simulink model "TwoDofPassengerCarModel"  (R2021b)
settings: Solver=VariableStepAuto  StartTime=0.0  StopTime=30  RelTol=1e-3
PreLoadFcn:
  | clearvars;
  | M1=300;
  | M2=30;
  | K1=10000;
  | K2=50000;
  | b1=100;
  | b2=30000;
settings Model: Creator=adish  LastModifiedBy=adish

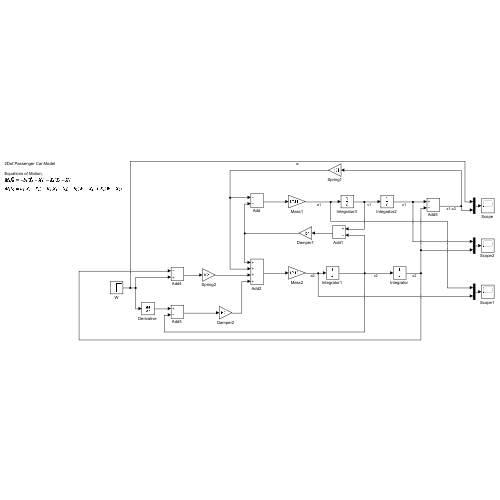
[thumbnail: Simulink's stored preview of the top-level diagram]
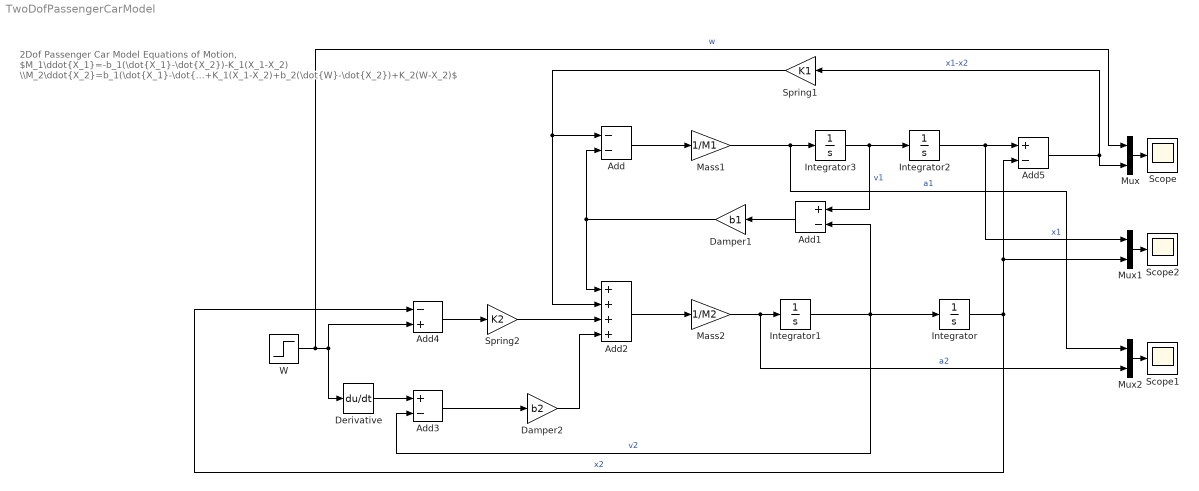
== system TwoDofPassengerCarModel ==
  note: 2Dof Passenger Car Model
      |
      | Equations of Motion,
      | $M_1\ddot{X_1}=-b_1(\dot{X_1}-\dot{X_2})-K_1(X_1-X_2) \\M_2\ddot{X_2}=b_1(\dot{X_1}-\dot{X_2})+K_1(X_1-X_2)+b_2(\dot{W}-\dot{X_2})+K_2(W-X_2)$
  "Add " : Sum  Inputs=--
  "Add1 " : Sum  Inputs=+-
  "Add2 " : Sum  Inputs=++++
  "Add3 " : Sum  Inputs=+-
  "Add4 " : Sum  Inputs=-+
  "Add5 " : Sum  Inputs=+-
  Damper1 : Gain  Gain=b1
  Damper2 : Gain  Gain=b2
  "Derivative " : Derivative
  "Integrator " : Integrator
  "Integrator1 " : Integrator
  "Integrator2 " : Integrator
  "Integrator3 " : Integrator
  Mass1 : Gain  Gain=1/M1
  Mass2 : Gain  Gain=1/M2
  Mux : Mux  Inputs=2
  Mux1 : Mux  Inputs=2
  Mux2 : Mux  Inputs=2
  "Scope " : Scope
  "Scope1 " : Scope
  "Scope2 " : Scope
  Spring1 : Gain  Gain=K1
  Spring2 : Gain  Gain=K2
  W : Step  SampleTime=0.05
  wires:
  W/1 -> Mux/1, "Add4 "/2, "Derivative "/1  "w"
  "Derivative "/1 -> "Add3 "/1
  "Add3 "/1 -> Damper2/1
  "Add4 "/1 -> Spring2/1
  Spring2/1 -> "Add2 "/3
  Damper2/1 -> "Add2 "/4
  "Add2 "/1 -> Mass2/1
  Mass2/1 -> Mux2/2, "Integrator1 "/1  "a2"
  "Integrator1 "/1 -> "Add3 "/2, "Add1 "/2, "Integrator "/1  "v2"
  "Integrator "/1 -> Mux1/2, "Add5 "/2, "Add4 "/1  "x2"
  "Integrator2 "/1 -> Mux1/1, "Add5 "/1  "x1"
  "Add5 "/1 -> Mux/2, Spring1/1  "x1-x2"
  "Add1 "/1 -> Damper1/1
  "Integrator3 "/1 -> "Add1 "/1, "Integrator2 "/1  "v1"
  Mass1/1 -> Mux2/1, "Integrator3 "/1  "a1"
  "Add "/1 -> Mass1/1
  Damper1/1 -> "Add "/2, "Add2 "/1
  Spring1/1 -> "Add2 "/2, "Add "/1
  Mux/1 -> "Scope "/1
  Mux1/1 -> "Scope2 "/1
  Mux2/1 -> "Scope1 "/1
